simulink model "househeat_single_param_issue"  (R2015b)
settings: Solver=ode45  StartTime=0.0  StopTime=24  RelTol=1e-3
model workspace (MAT data in the model file):
  M_heater_air = 3600
  R_equivalent = 4.329e-07
  STOICAL.LabelDefinition.Hierarchical = {'#UNIT#'}
  STOICAL.LabelDefinition.Signals = {'#SIG#'}
  STOICAL.LabelDefinition.Parameters = {'#PARAM#'}
  STOICAL.LabelDefinition.DefaultVariant = {'#DEF#'}
  STOICAL.SignalSaveOptions.ReturnWorkspaceOutputs = 'on'
  STOICAL.SignalSaveOptions.ReturnWorkspaceOutputsName = 'simout_obj'
  STOICAL.SignalSaveOptions.SignalLogging = 'on'
  STOICAL.SignalSaveOptions.SignalLoggingSaveFormat = 'Dataset'
  STOICAL.SignalSaveOptions.SignalLoggingName = 'STOICAL_LoggedSignals'
  STOICAL.ParameterDefinition.NrParams = 0
  STOICAL.ParameterDefinition.BlkField2Set = {''}
  STOICAL.ParameterDefinition.BlkFieldSyntax = {''}
  STOICAL.ParameterDefinition.LabelPath = {}
  STOICAL.ParameterDefinition.ParamDefaultValue = {}
  STOICAL.SignalDefinition.ParentalBlockPath = {''}
  STOICAL.SignalDefinition.ParentalBlockHandle = {}
  STOICAL.SignalDefinition.NameInDiagram = {}
  STOICAL.SignalDefinition.SourceBlockPath = {''}
  STOICAL.SignalDefinition.SourceBlockPort = {}
  STOICAL.SignalDefinition.SourceBlockHandle = {}
  STOICAL.SignalDefinition.Handle = []
  STOICAL.SignalDefinition.NrSig = 0
  STOICAL.SignalDefinition.NameOfLogVar = {}
  STOICAL.SignalDefinition.NameOfLogVarMode = {}
  STOICAL.SignalDefinition.DoLog = []
  STOICAL.SignalDefinition.LabelPath = {''}
  STOICAL.VariantDefinition.NodeHandle = [93.0015869141; 96.0017089844; 2081.00036621; 2099.00036621; 2107.00036621]
  STOICAL.VariantDefinition.NodeName = {'househeat_single_param_issue'; 'Heater'; 'Room'; 'Signal Builder'; 'Thermostat'}
  STOICAL.VariantDefinition.IsVariantSubsystem = [0; 0; 0; 0; 0]
  STOICAL.VariantDefinition.NodeLevel = [1; 2; 2; 2; 2]
  STOICAL.VariantDefinition.NodePath = {'househeat_single_param_issue'; 'househeat_single_param_issue/Heater'; 'househeat_single_param_issue/Room'; 'househeat_single_param_issue/Signal Builder'; 'househeat_single_param_issue/Thermostat'}
  STOICAL.VariantDefinition.IsVariant = [0; 0; 0; 0; 0]
  STOICAL.VariantDefinition.VSNodeIdxofVariant = [0; 0; 0; 0; 0]
  STOICAL.VariantDefinition.VSVariantsCount = [0; 0; 0; 0; 0]
  STOICAL.VariantDefinition.VSVariantsBlkHdls = {[]; []; []; []; []}
  STOICAL.VariantDefinition.VSVariantsNodeIdx = {[]; []; []; []; []}
  STOICAL.VariantDefinition.VSControlVariable = {[]; []; []; []; []}
  STOICAL.VariantDefinition.VSVariantHasNr = [0; 0; 0; 0; 0]
  STOICAL.VariantDefinition.LabelPath = {[]; []; []; []; []}
  T_heater = 50
  T_roomIC = 20
  c_air = 1005.4
  m_room_air = 1470
undefined symbols (not defined in the file): sigbuilder_block, TempSoll
settings Model: Creator=homann  LastModifiedBy=homann
settings DataIOCC: SaveOutput=off  InspectSignalLogs=on  VisualizeSimOutput=off  SaveTime=off  ReturnWorkspaceOutputs=on  SignalLoggingName=STOICAL_LoggedSignals  ReturnWorkspaceOutputsName=simout_obj

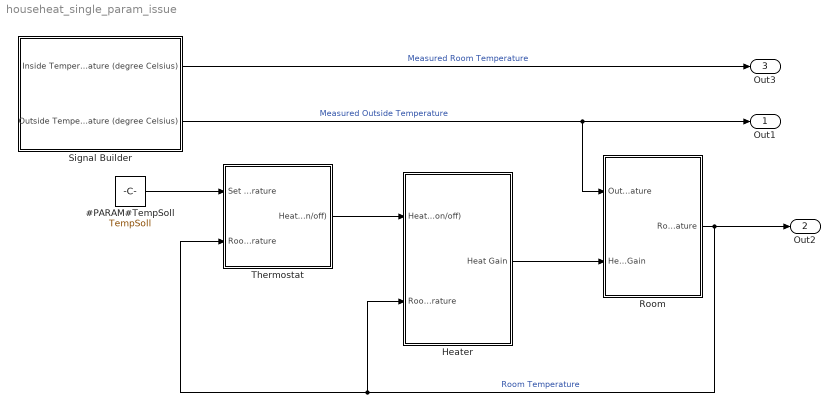
== system househeat_single_param_issue ==
  #PARAM#TempSoll : Constant  Value=TempSoll
  Heater : Subsystem
  Room : Subsystem
  Signal Builder : Subsystem  Tag=STV Subsys  LoadFcn=sigbuilder_block('load');  StartFcn=sigbuilder_block('start');  StopFcn=sigbuilder_block('stop');  ClipboardFcn=sigbuilder_block('clipboard');  mask(Sigbuilder block){}
      mask help: Simulink:masks:SigbuilderBlock_MD
      mask init:
      | if ~strcmp(get_param(bdroot(gcbh),'SimulationStatus'),'stopped') tuvar = sigbuilder_block('maskInit'); end
      settings: CopyFcn=sigbuilder_block('copy');  DeleteFcn=sigbuilder_block('delete');  ModelCloseFcn=sigbuilder_block('modelClose');  PreSaveFcn=sigbuilder_block('preSave');  PauseFcn=sigbuilder_block('pause');  ContinueFcn=sigbuilder_block('continue');  NameChangeFcn=sigbuilder_block('namechange');  OpenFcn=sigbuilder_block('open',[437.6 199.2 550.4 400 ]);  CloseFcn=sigbuilder_block('close');
      mask Display: plot(0, 0, 100, 100,[2, 2, 32, 32, 2], [68, 8, 8, 68, 68],[32, 2], [38, 38], [32, 19, 2],[53, 60, 44], [32, 17, 17, 2],[16, 16, 31, 31]);txt = getActiveGroup(gcbh);text(2, 100, txt,'verticalAlignment', 'top');
  Thermostat : Subsystem
  Out1 : Outport
  Out2 : Outport  Port=2
  Out3 : Outport  Port=3
  wires:
  Thermostat/1(Heater (on/off)) -> Heater/1(Heater (on/off))
  Room/1(Room Temperature) -> Heater/2(Room Temperature), Thermostat/2(Room Temperature), Out2/1  "Room Temperature"
  Heater/1(Heat Gain) -> Room/2(Heat Gain)
  #PARAM#TempSoll/1 -> Thermostat/1(Set Room Temperature)
  Signal Builder/2(Outside Temperature (degree Celsius)) -> Room/1(Outside Temperature), Out1/1  "Measured Outside Temperature"
  Signal Builder/1(Inside Temperature (degree Celsius)) -> Out3/1  "Measured Room Temperature"

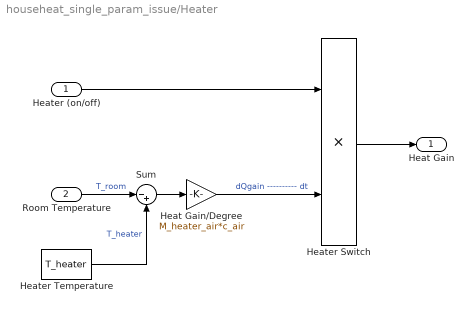
== system househeat_single_param_issue/Heater ==
  Heater (on/off) : Inport
  Room Temperature : Inport  Port=2
  Heat Gain/Degree : Gain  Gain=M_heater_air*c_air
  Heater Switch : Product
  Heater Temperature : Constant  Value=T_heater
  Sum : Sum  Inputs=|-+
  Heat Gain : Outport
  wires:
  Heater Temperature/1 -> Sum/2  "T_heater"
  Room Temperature/1 -> Sum/1  "T_room"
  Sum/1 -> Heat Gain/Degree/1
  Heater (on/off)/1 -> Heater Switch/1
  Heater Switch/1 -> Heat Gain/1
  Heat Gain/Degree/1 -> Heater Switch/2  "dQgain ---------- dt"

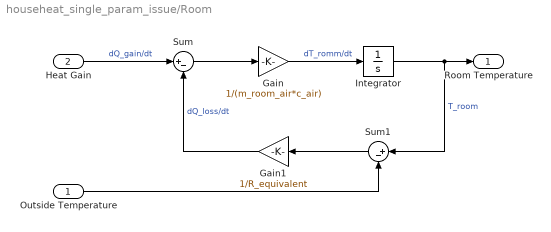
== system househeat_single_param_issue/Room ==
  Outside Temperature : Inport
  Heat Gain : Inport  Port=2
  Gain : Gain  Gain=1/(m_room_air*c_air)
  Gain1 : Gain  Gain=1/R_equivalent
  Integrator : Integrator  InitialCondition=T_roomIC
  Sum : Sum  Inputs=|+-
  Sum1 : Sum  Inputs=|+-
  Room Temperature : Outport
  wires:
  Heat Gain/1 -> Sum/1  "dQ_gain/dt"
  Gain1/1 -> Sum/2  "dQ_loss/dt"
  Sum/1 -> Gain/1
  Gain/1 -> Integrator/1  "dT_romm/dt"
  Integrator/1 -> Sum1/1, Room Temperature/1  "T_room"
  Outside Temperature/1 -> Sum1/2
  Sum1/1 -> Gain1/1

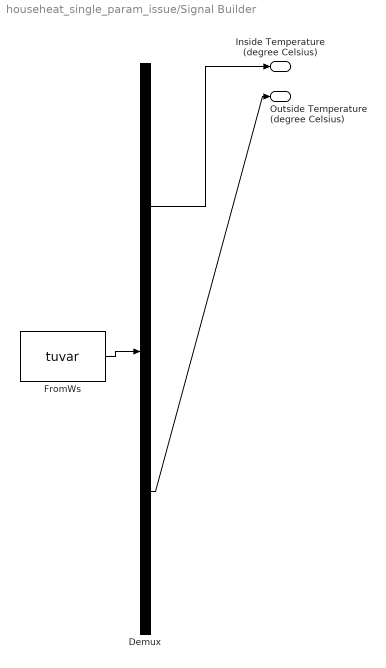
== system househeat_single_param_issue/Signal Builder ==
  Demux : Demux  Tag=STV Demux  Outputs=2
  FromWs : FromWorkspace  Tag=STV FromWs  VariableName=tuvar  SampleTime=0
      SigBuilderData=|
      | common.afterFinalStr = 'Extrapolate'
      | common.sampleTime = 0
      | dataSet.timeRange = [0 23.9]
      | dataSet.name = 'Measured Data'
      | sbobj.Name = 'Signal Builder'
      | sbobj.Groups.Name = 'Measured Data'
      | sbobj.Groups.Signals(1).Name = 'Inside Temperature (degree Celsius)'
      | sbobj.Groups.Signals(1).XData = [0 0.1 0.2 0.3 0.4 0.5 0.6 0.7 0.8 0.9 1 1.1 1.2 1.3 1.4 1.5 1.6 1.7 1.8 1.9 2 2.1 2.2 2.3 2.4 2.5 2.6 2.7 2.8 2.9 3 3.1 3.2 3.3 3.4 3.5 3.6 3.7 3.8 3.9 4 4.1 4.2 4.3 4.4 4.5 4.6 4.7 4.8 4.9 5 5.1 5.2 5.3 5.4 5.5 5.6 5.7 5.8 5.9 6 6.1 6.2 6.3 6.4 6.5 6.6 6.7 6.8 6.9 7 7.1 7.2 7.3 7.4 7.5 7.6 7.7 7.8 7.9 8 8.1 8.2 8.3 8.4 8.5 8.6 8.7 8.8 8.9 9 9.1 9.2 9.3 9.4 9.5 9.6 9.7 9.8 9.9 10 10.1 10.2 10.3 10.4 10.5 10.6 10.7 10.8 10.9 11 11.1 11.2 11.3 11.4 11.5 11.6 11.7 11.8 11.9 12 12.1 12.2 12.3 12.4 12.5 12.6 12.7 12.8 12.9 13 13.1 13.2 13.3 13.4 13.5 13.6 13.7 13.8 13.9 14 14.1 14.2 14.3 14.4 14.5 14.6 14.7 14.8 14.9 15 15.1 15.2 15.3 15.4 15.5 15.6 15.7 15.8 15.9 16 16.1 16.2 16.3 16.4 16.5 16.6 16.7 16.8 16.9 17 17.1 17.2 17.3 17.4 17.5 17.6 17.7 17.8 17.9 18 18.1 18.2 18.3 18.4 18.5 18.6 18.7 18.8 18.9 19 19.1 19.2 19.3 19.4 19.5 19.6 19.7 19.8 19.9 20 20.1 20.2 20.3 20.4 20.5 20.6 20.7 20.8 20.9 21 21.1 21.2 21.3 21.4 21.5 21.6 21.7 21.8 21.9 22 22.1 22.2 22.3 22.4 22.5 22.6 22.7 22.8 22.9 23 23.1 23.2 23.3 23.4 23.5 23.6 23.7 23.8 23.9]
      | sbobj.Groups.Signals(1).YData = [25.2 21 20 19.7 24.6 25.3 21.3 19.6 22.8 25.7 23.2 20.6 19.8 22.5 24.5 22.4 20.6 19.7 22.1 25.2 22.5 20.3 19.7 24.6 25.8 22 20.3 19.8 24.9 23.5 21.2 19.7 23.6 25.4 22.1 20.5 19.8 25.1 23.2 21 19.8 22.8 24.5 20.6 19.8 22.7 25.2 22.4 20.7 20.2 19.9 25.2 23.1 21 20.2 19.6 23.4 25.4 22.1 20.6 19.8 22.5 25.2 22.6 20.8 19.9 19.5 22.6 25.5 22.9 21 19.7 23.1 25.6 23.2 20.9 20 19.5 21.3 25.5 22.8 20.6 19.8 19.5 23.6 25.3 22.1 20.5 19.5 20.4 24.9 21.4 20.2 19.9 19.6 20.4 24.7 21.8 20.6 20.4 20.3 20.1 20.1 20.2 20.2 20.2 20.3 20.3 20.4 20.4 20.5 20.6 20.5 20.4 20.5 20.6 20.8 20.8 20.6 20.7 20.8 20.9 21.2 21.1 21.2 21.3 21.3 21.3 21.4 21.5 21.5 21.5 21.6 21.7 21.8 21.8 21.9 21.8 21.9 21.9 21.9 22 22 21.9 22 22.1 22.1 22 22.1 22.1 22.1 22.2 22.1 22.1 22.1 22 22 21.9 21.8 21.9 21.8 21.7 21.7 21.6 21.6 21.5 21.5 21.3 21.3 21.2 21.1 21.1 21 20.8 20.9 20.9 20.8 20.7 20.6 20.6 20.5 20.4 20.4 20.4 20.3 20.3 20.2 20.2 20 19.9 19.8 19.6 21.3 23 24.8 21 20.5 20.2 20 19.8 24.2 25 21 20 19.8 19.8 21.6 25.1 21.6 20.3 19.8 19.7 25 22.3 20.8 20 19.7 19.5 25.5 22.8 21 20.3 19.8 19.4 23.8 25.2 21.7 20 19.6 22 25.3 21.7 20.1 20 23 25.3 21.7 20.2 19.7 24.1]
      | sbobj.Groups.Signals(2).Name = 'Outside Temperature (degree Celsius)'
      | sbobj.Groups.Signals(2).XData = [0 0.1 0.2 0.3 0.4 0.5 0.6 0.7 0.8 0.9 1 1.1 1.2 1.3 1.4 1.5 1.6 1.7 1.8 1.9 2 2.1 2.2 2.3 2.4 2.5 2.6 2.7 2.8 2.9 3 3.1 3.2 3.3 3.4 3.5 3.6 3.7 3.8 3.9 4 4.1 4.2 4.3 4.4 4.5 4.6 4.7 4.8 4.9 5 5.1 5.2 5.3 5.4 5.5 5.6 5.7 5.8 5.9 6 6.1 6.2 6.3 6.4 6.5 6.6 6.7 6.8 6.9 7 7.1 7.2 7.3 7.4 7.5 7.6 7.7 7.8 7.9 8 8.1 8.2 8.3 8.4 8.5 8.6 8.7 8.8 8.9 9 9.1 9.2 9.3 9.4 9.5 9.6 9.7 9.8 9.9 10 10.1 10.2 10.3 10.4 10.5 10.6 10.7 10.8 10.9 11 11.1 11.2 11.3 11.4 11.5 11.6 11.7 11.8 11.9 12 12.1 12.2 12.3 12.4 12.5 12.6 12.7 12.8 12.9 13 13.1 13.2 13.3 13.4 13.5 13.6 13.7 13.8 13.9 14 14.1 14.2 14.3 14.4 14.5 14.6 14.7 14.8 14.9 15 15.1 15.2 15.3 15.4 15.5 15.6 15.7 15.8 15.9 16 16.1 16.2 16.3 16.4 16.5 16.6 16.7 16.8 16.9 17 17.1 17.2 17.3 17.4 17.5 17.6 17.7 17.8 17.9 18 18.1 18.2 18.3 18.4 18.5 18.6 18.7 18.8 18.9 19 19.1 19.2 19.3 19.4 19.5 19.6 19.7 19.8 19.9 20 20.1 20.2 20.3 20.4 20.5 20.6 20.7 20.8 20.9 21 21.1 21.2 21.3 21.4 21.5 21.6 21.7 21.8 21.9 22 22.1 22.2 22.3 22.4 22.5 22.6 22.7 22.8 22.9 23 23.1 23.2 23.3 23.4 23.5 23.6 23.7 23.8 23.9]
      | sbobj.Groups.Signals(2).YData = [6.8 6.7 6.6 6.6 6.6 6.8 6.6 6.5 6.7 6.3 6.4 6.5 6.6 6.5 6.5 6.5 6.3 6.5 6.5 6.3 6 6.2 6.1 6 6 6 6.1 6.1 5.8 5.6 5.8 5.9 5.9 5.8 5.8 5.7 5.8 5.9 5.8 5.7 5.6 5.6 5.7 5.7 5.7 5.5 5.6 5.8 5.8 5.5 5.5 5.4 5.8 5.5 5.6 5.4 5.3 5.5 5.6 5.4 5.6 5.6 5.6 5.3 5.3 5.5 5.5 5.5 5.5 5.7 5.8 5.8 6.3 6.5 6.5 6.6 6.9 7.5 7.4 7.5 8.4 8.8 10.7 11 11.1 11.5 11.7 12.5 13.3 14 14.8 15 15.5 16.1 16.4 16.6 16.6 16.9 17.2 17.6 17.7 17.7 17.9 18.6 18.8 19.2 19.4 19.5 19.2 19.4 19.8 19.8 20 20 20.1 20.3 20.2 20 20.2 20.4 20.1 20.3 20.1 20.1 20.2 20.3 20.3 20.5 20.4 20.3 20.4 20.3 20.4 20.6 20.4 20.3 20.3 20.2 20.2 20.2 20.2 20.1 19.9 20 19.9 19.9 19.8 19.7 19.7 19.7 19.4 19.5 19.4 19.3 19.3 19.3 19.2 19.3 19 18.9 18.9 18.8 18.5 18.4 18 17.4 17.2 17 16.9 16.5 16.2 15.9 15.6 15.6 15.3 14.6 14 13.8 13.6 13.4 13.2 13 13 12.6 12.6 12.4 11.8 11.5 11.4 11.5 10.8 10.6 10.6 10.5 10.6 10.3 10.2 10.2 10 9.8 9.7 9.5 9.6 9.5 9.4 9.2 9 9.1 9.2 8.7 8.6 8.9 8.5 8.4 8.2 8.5 8.2 8.2 8 8 7.8 7.8 7.6 7.7 7.2 7.3 7.4 7.5 7 7 7.1 7.1 7.3 7.2 7 6.8 6.8 6.6 7 6.7]
      | sbobj.Groups.TimeRange = [0 23.9]
  Inside Temperature (degree Celsius) : Outport
  Outside Temperature (degree Celsius) : Outport  Tag=STV Outport  Port=2
  wires:
  Demux/1 -> Inside Temperature (degree Celsius)/1
  FromWs/1 -> Demux/1
  Demux/2 -> Outside Temperature (degree Celsius)/1

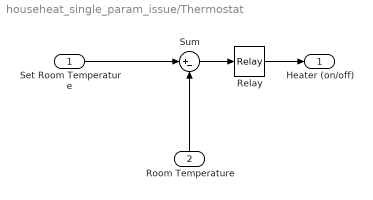
== system househeat_single_param_issue/Thermostat ==
  Set Room Temperature : Inport
  Room Temperature : Inport  Port=2
  Relay : Relay  OnSwitchValue=0  OffSwitchValue=-5
  Sum : Sum  Inputs=|+-
  Heater (on/off) : Outport
  wires:
  Set Room Temperature/1 -> Sum/1
  Room Temperature/1 -> Sum/2
  Sum/1 -> Relay/1
  Relay/1 -> Heater (on/off)/1
